simulink model "velocity_test"  (R2019b)
settings: Solver=VariableStepAuto  StartTime=0.0  StopTime=10.0  RelTol=1e-3
libraries: drivinglib x1
settings Model: Creator=Gautam Gupta  LastModifiedBy=Gautam Gupta

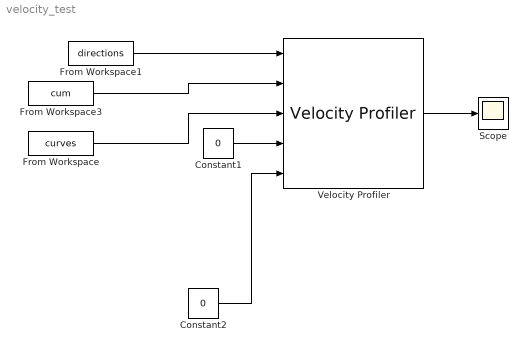
== system velocity_test ==
  Constant1 : Constant  Value=0
  Constant2 : Constant  Value=0
  From Workspace : FromWorkspace  VariableName=curves  SampleTime=0
  From Workspace1 : FromWorkspace  VariableName=directions  SampleTime=0
  From Workspace3 : FromWorkspace  VariableName=cum  SampleTime=0
  Scope : Scope
  Velocity Profiler : drivinglib/Velocity Profiler  MaxLongitudinalAccel=3  MaxLongitudinalDecel=6  MaxSpeed=10  MaxLongitudinalJerk=1  MaxLateralAccel=1  ShowOptionalOutport=off  SampleTime=-1  SimulateUsing=Code generation
      settings: SourceProductName=Automated Driving Toolbox  SourceProductBaseCode=DR
  wires:
  From Workspace/1 -> Velocity Profiler/3
  From Workspace3/1 -> Velocity Profiler/2
  From Workspace1/1 -> Velocity Profiler/1
  Constant1/1 -> Velocity Profiler/4
  Constant2/1 -> Velocity Profiler/5
  Velocity Profiler/1 -> Scope/1
